simulink model "model_filters"  (R2018a)
settings: Solver=VariableStepAuto  StartTime=0.0  StopTime=6  RelTol=1e-3
PreLoadFcn:
  | load('alberto_data.mat')
model workspace (MAT data in the model file):
  fc = Simulink.Parameter
  fc.Value = 300
  fc.DataType = 'auto'
  fc.Dimensions = [1 1]
settings Model: Creator=stefanobuccelli  LastModifiedBy=stefanobuccelli

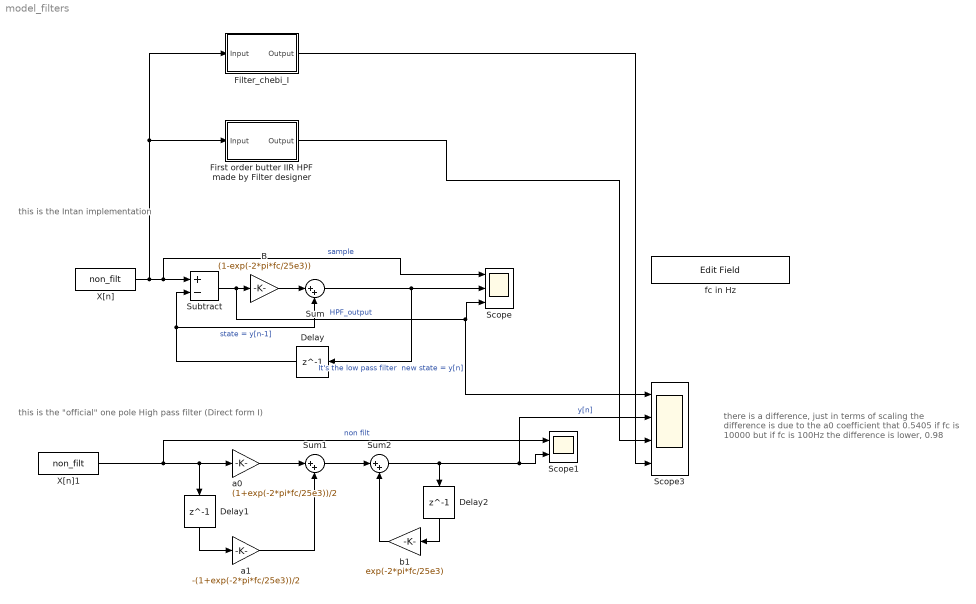
== system model_filters ==
  note: this is the "official" one pole High pass filter (Direct form I)
  note: this is the Intan implementation
  note: there is a difference, just in terms of scaling
      | the difference is due to the a0 coefficient that 0.5405
      | if fc is 10000 but if fc is 100Hz the
      | difference is lower, 0.98
  B : Gain  Gain=(1-exp(-2*pi*fc/25e3))
  Delay : Delay  DelayLength=1
  Delay1 : Delay  DelayLength=1
  Delay2 : Delay  DelayLength=1
  Filter_chebi_I : Subsystem  Tag=FilterWizardSubSystem
      settings: ErrorFcn=dspFilterRealizedInBasicElemsAlgLoopErrFcnCallback
  First order butter IIR HPF made by Filter designer : Subsystem  Tag=FilterWizardSubSystem
      settings: ErrorFcn=dspFilterRealizedInBasicElemsAlgLoopErrFcnCallback
  Scope : Scope  NumInputPorts=3
  Scope1 : Scope  NumInputPorts=2
  Scope3 : Scope  NumInputPorts=4
  Subtract : Sum  Inputs=+-
  Sum : Sum  Inputs=|++
  Sum1 : Sum  Inputs=|++
  Sum2 : Sum  Inputs=|++
  X[n] : FromWorkspace  VariableName=non_filt  SampleTime=1/25e3  OutputAfterFinalValue=Setting to zero
  X[n]1 : FromWorkspace  VariableName=non_filt  SampleTime=1/25e3  OutputAfterFinalValue=Holding final value
  a0 : Gain  Gain=(1+exp(-2*pi*fc/25e3))/2
  a1 : Gain  Gain=-(1+exp(-2*pi*fc/25e3))/2
  b1 : Gain  Gain=exp(-2*pi*fc/25e3)
  fc in Hz : EditField  WebBlockId=206  LabelPosition=Hide  Alignment=Center
  wires:
  X[n]/1 -> First order butter IIR HPF made by Filter designer/1(Input), Filter_chebi_I/1(Input), Scope/1, Subtract/1  "sample"
  Subtract/1 -> Scope3/1, Scope/3, B/1  "HPF_output"
  B/1 -> Sum/1
  Sum/1 -> Delay/1, Scope/2  "It's the low pass filter  new state = y[n]"
  Delay/1 -> Sum/2, Subtract/2  "state = y[n-1]"
  X[n]1/1 -> a0/1, Delay1/1, Scope1/1  "non filt"
  a1/1 -> Sum1/2
  Sum2/1 -> Scope3/2, Scope1/2, Delay2/1  "y[n]"
  Sum1/1 -> Sum2/1
  Delay1/1 -> a1/1
  Delay2/1 -> b1/1
  b1/1 -> Sum2/2
  a0/1 -> Sum1/1
  First order butter IIR HPF made by Filter designer/1(Output) -> Scope3/3
  Filter_chebi_I/1(Output) -> Scope3/4

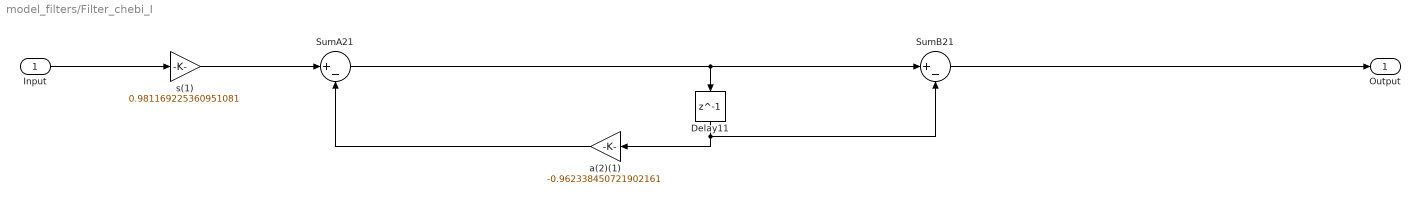
== system model_filters/Filter_chebi_I ==
  Input : Inport
  Delay11 : Delay  DelayLength=1  InitialCondition=0
  SumA21 : Sum  Inputs=|+-  RndMeth=Nearest  SaturateOnIntegerOverflow=on  OutDataTypeStr=Inherit: Same as first input
  SumB21 : Sum  Inputs=|+-  RndMeth=Nearest  SaturateOnIntegerOverflow=on  OutDataTypeStr=Inherit: Same as first input
  a(2)(1) : Gain  Gain=-0.962338450721902161  ParamDataTypeStr=double  RndMeth=Nearest  SaturateOnIntegerOverflow=on  OutDataTypeStr=Inherit: Same as input
  s(1) : Gain  Gain=0.981169225360951081  ParamDataTypeStr=double  RndMeth=Nearest  SaturateOnIntegerOverflow=on  OutDataTypeStr=Inherit: Same as input
  Output : Outport
  wires:
  Input/1 -> s(1)/1
  s(1)/1 -> SumA21/1
  SumA21/1 -> SumB21/1, Delay11/1
  SumB21/1 -> Output/1
  a(2)(1)/1 -> SumA21/2
  Delay11/1 -> a(2)(1)/1, SumB21/2

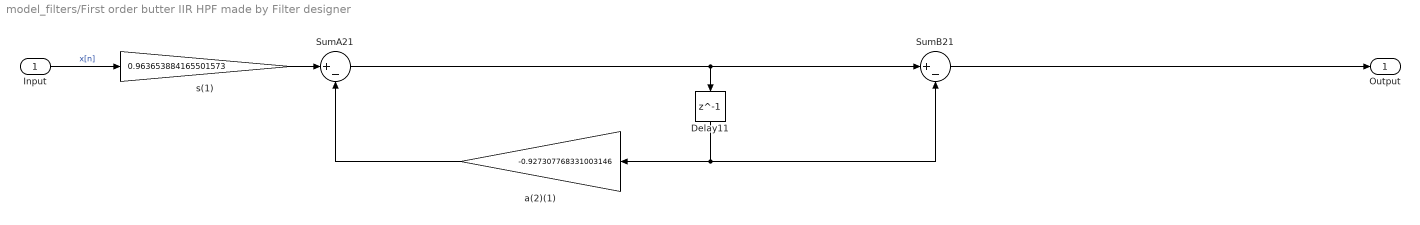
== system model_filters/First order butter IIR HPF made by Filter designer ==
  Input : Inport
  Delay11 : Delay  DelayLength=1  InitialCondition=0
  SumA21 : Sum  Inputs=|+-  RndMeth=Nearest  SaturateOnIntegerOverflow=on  OutDataTypeStr=Inherit: Same as first input
  SumB21 : Sum  Inputs=|+-  RndMeth=Nearest  SaturateOnIntegerOverflow=on  OutDataTypeStr=Inherit: Same as first input
  a(2)(1) : Gain  Gain=-0.927307768331003146  ParamDataTypeStr=double  RndMeth=Nearest  SaturateOnIntegerOverflow=on  OutDataTypeStr=Inherit: Same as input
  s(1) : Gain  Gain=0.963653884165501573  ParamDataTypeStr=double  RndMeth=Nearest  SaturateOnIntegerOverflow=on  OutDataTypeStr=Inherit: Same as input
  Output : Outport
  wires:
  Input/1 -> s(1)/1  "x[n]"
  s(1)/1 -> SumA21/1
  SumA21/1 -> SumB21/1, Delay11/1
  SumB21/1 -> Output/1
  a(2)(1)/1 -> SumA21/2
  Delay11/1 -> a(2)(1)/1, SumB21/2
